simulink model "Q43_sim"  (R2023a)
settings: Solver=FixedStepAuto  StartTime=0.0  StopTime=5  FixedStep=0.001  RelTol=1e-3
values from neighbouring files (symbols this model uses):
  Ca_ld = -k_a_ld*tf([tao_a_ld 1],[alpha_a_ld*tao_a_ld 1])    [PreLab3_script.m]
  Cp_ld = k_ld*tf([tao_ld 1],[alpha_ld*tao_ld 1])    [PreLab3_script.m]
  Cp_PI = Cp_PI_no_Kp*Kp    [PreLab3_script.m]
  G1 = tf([K_gain1 0],1) * (tf(1,[1 -p1]) * tf(1,[1 -p2]) * tf(1,[1 -p3]))    [PreLab3_script.m]
  G2 = (K_gain2 * tf([1 -z1],1) * tf([1 -z2],1)) * (tf(1,[1 -p1]) * tf(1,[1 -p2]) * tf(1,[1 -p3]))*tf(1,[1 0])    [PreLab3_script.m]
settings Model: Creator=אלמוג  LastModifiedBy=אלמוג

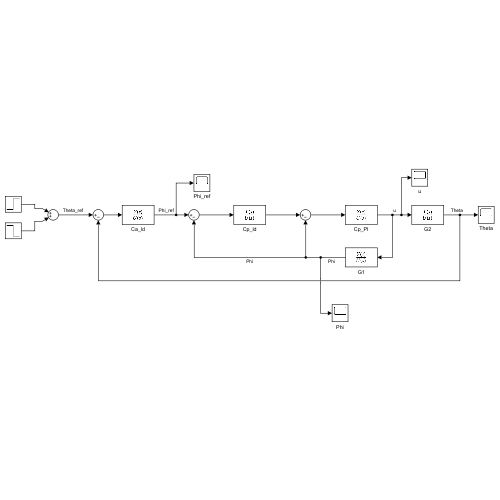
[thumbnail: Simulink's stored preview of the top-level diagram]
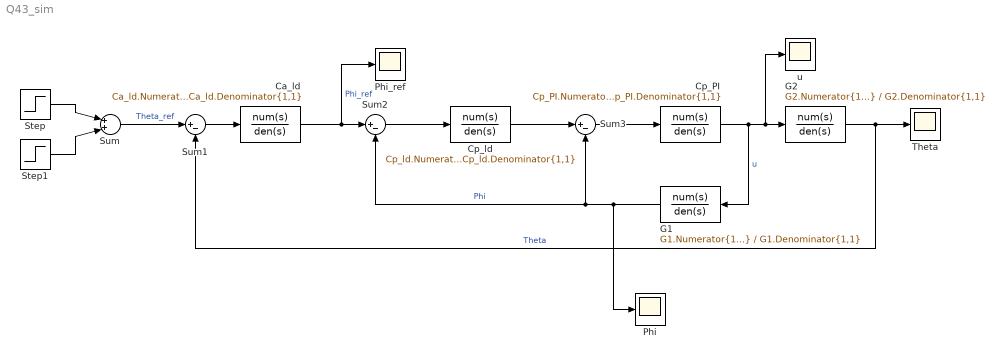
== system Q43_sim ==
  Ca_ld : TransferFcn  Numerator=Ca_ld.Numerator{1,1}  Denominator=Ca_ld.Denominator{1,1}
  Cp_PI : TransferFcn  Numerator=Cp_PI.Numerator{1,1}  Denominator=Cp_PI.Denominator{1,1}
  Cp_ld : TransferFcn  Numerator=Cp_ld.Numerator{1,1}  Denominator=Cp_ld.Denominator{1,1}
  G1 : TransferFcn  Numerator=G1.Numerator{1,1}  Denominator=G1.Denominator{1,1}
  G2 : TransferFcn  Numerator=G2.Numerator{1,1}  Denominator=G2.Denominator{1,1}
  Phi : Scope
  Phi_ref : Scope
  Step : Step  Time=0.1  After=pi/10  SampleTime=0
  Step1 : Step  Time=0.2  After=-pi/10  SampleTime=0
  Sum : Sum  Inputs=|++|
  Sum1 : Sum  Inputs=|+-
  Sum2 : Sum  Inputs=|+-
  Sum3 : Sum  Inputs=|+-
  Theta : Scope
  u : Scope
  wires:
  Step1/1 -> Sum/2
  Step/1 -> Sum/1
  Sum/1 -> Sum1/1  "Theta_ref"
  Sum1/1 -> Ca_ld/1
  Ca_ld/1 -> Phi_ref/1, Sum2/1  "Phi_ref"
  Sum2/1 -> Cp_ld/1
  Cp_ld/1 -> Sum3/1
  Sum3/1 -> Cp_PI/1
  Cp_PI/1 -> G1/1, u/1, G2/1  "u"
  G1/1 -> Phi/1, Sum2/2, Sum3/2  "Phi"
  G2/1 -> Sum1/2, Theta/1  "Theta"
